simulink model "test_mdl_NI"  (R2018a)
settings: Solver=VariableStepAuto  StartTime=0.0  StopTime=10.0  RelTol=1e-3
(part 24 of 24)

== system test_mdl_NI/To_NI_HIL/SRR_L/RL_SOD/SRR_RL_002/SRR_RL_CAN_DET_RANGE_02 ==
  in : Inport
  out : Outport
  wires:
  in/1 -> out/1

== system test_mdl_NI/To_NI_HIL/SRR_L/RL_SOD/SRR_RL_002/SRR_RL_CAN_DET_RANGE_RATE_02 ==
  in : Inport
  out : Outport
  wires:
  in/1 -> out/1

== system test_mdl_NI/To_NI_HIL/SRR_L/RL_SOD/SRR_RL_002/SRR_RL_CAN_DET_SUPER_RES_TARGET_02 ==
  in : Inport
  out : Outport
  wires:
  in/1 -> out/1

== system test_mdl_NI/To_NI_HIL/SRR_L/RL_SOD/SRR_RL_002/SRR_RL_CAN_DET_VALID_LEVEL_02 ==
  in : Inport
  out : Outport
  wires:
  in/1 -> out/1

== system test_mdl_NI/To_NI_HIL/SRR_L/RL_SOD/SRR_RL_003/SRR_RL_CAN_DET_AMPLITUDE_03 ==
  in : Inport
  out : Outport
  wires:
  in/1 -> out/1

== system test_mdl_NI/To_NI_HIL/SRR_L/RL_SOD/SRR_RL_003/SRR_RL_CAN_DET_AZIMUTH_03 ==
  in : Inport
  out : Outport
  wires:
  in/1 -> out/1

== system test_mdl_NI/To_NI_HIL/SRR_L/RL_SOD/SRR_RL_003/SRR_RL_CAN_DET_ELEVATION_03 ==
  in : Inport
  out : Outport
  wires:
  in/1 -> out/1

== system test_mdl_NI/To_NI_HIL/SRR_L/RL_SOD/SRR_RL_003/SRR_RL_CAN_DET_RANGE_03 ==
  in : Inport
  out : Outport
  wires:
  in/1 -> out/1

== system test_mdl_NI/To_NI_HIL/SRR_L/RL_SOD/SRR_RL_003/SRR_RL_CAN_DET_RANGE_RATE_03 ==
  in : Inport
  out : Outport
  wires:
  in/1 -> out/1

== system test_mdl_NI/To_NI_HIL/SRR_L/RL_SOD/SRR_RL_003/SRR_RL_CAN_DET_SUPER_RES_TARGET_03 ==
  in : Inport
  out : Outport
  wires:
  in/1 -> out/1

== system test_mdl_NI/To_NI_HIL/SRR_L/RL_SOD/SRR_RL_003/SRR_RL_CAN_DET_VALID_LEVEL_03 ==
  in : Inport
  out : Outport
  wires:
  in/1 -> out/1

== system test_mdl_NI/To_NI_HIL/SRR_R/FR_SOD/SRR_FR_001/SRR_FR_CAN_DET_AMPLITUDE_01 ==
  in : Inport
  out : Outport
  wires:
  in/1 -> out/1

== system test_mdl_NI/To_NI_HIL/SRR_R/FR_SOD/SRR_FR_001/SRR_FR_CAN_DET_AZIMUTH_01 ==
  in : Inport
  out : Outport
  wires:
  in/1 -> out/1

== system test_mdl_NI/To_NI_HIL/SRR_R/FR_SOD/SRR_FR_001/SRR_FR_CAN_DET_ELEVATION_01 ==
  in : Inport
  out : Outport
  wires:
  in/1 -> out/1

== system test_mdl_NI/To_NI_HIL/SRR_R/FR_SOD/SRR_FR_001/SRR_FR_CAN_DET_RANGE_01 ==
  in : Inport
  out : Outport
  wires:
  in/1 -> out/1

== system test_mdl_NI/To_NI_HIL/SRR_R/FR_SOD/SRR_FR_001/SRR_FR_CAN_DET_RANGE_RATE_01 ==
  in : Inport
  out : Outport
  wires:
  in/1 -> out/1

== system test_mdl_NI/To_NI_HIL/SRR_R/FR_SOD/SRR_FR_001/SRR_FR_CAN_DET_SUPER_RES_TARGET_01 ==
  in : Inport
  out : Outport
  wires:
  in/1 -> out/1

== system test_mdl_NI/To_NI_HIL/SRR_R/FR_SOD/SRR_FR_001/SRR_FR_CAN_DET_VALID_LEVEL_01 ==
  in : Inport
  out : Outport
  wires:
  in/1 -> out/1

== system test_mdl_NI/To_NI_HIL/SRR_R/FR_SOD/SRR_FR_002/SRR_FR_CAN_DET_AMPLITUDE_02 ==
  in : Inport
  out : Outport
  wires:
  in/1 -> out/1

== system test_mdl_NI/To_NI_HIL/SRR_R/FR_SOD/SRR_FR_002/SRR_FR_CAN_DET_AZIMUTH_02 ==
  in : Inport
  out : Outport
  wires:
  in/1 -> out/1

== system test_mdl_NI/To_NI_HIL/SRR_R/FR_SOD/SRR_FR_002/SRR_FR_CAN_DET_ELEVATION_02 ==
  in : Inport
  out : Outport
  wires:
  in/1 -> out/1

== system test_mdl_NI/To_NI_HIL/SRR_R/FR_SOD/SRR_FR_002/SRR_FR_CAN_DET_RANGE_02 ==
  in : Inport
  out : Outport
  wires:
  in/1 -> out/1

== system test_mdl_NI/To_NI_HIL/SRR_R/FR_SOD/SRR_FR_002/SRR_FR_CAN_DET_RANGE_RATE_02 ==
  in : Inport
  out : Outport
  wires:
  in/1 -> out/1

== system test_mdl_NI/To_NI_HIL/SRR_R/FR_SOD/SRR_FR_002/SRR_FR_CAN_DET_SUPER_RES_TARGET_02 ==
  in : Inport
  out : Outport
  wires:
  in/1 -> out/1

== system test_mdl_NI/To_NI_HIL/SRR_R/FR_SOD/SRR_FR_002/SRR_FR_CAN_DET_VALID_LEVEL_02 ==
  in : Inport
  out : Outport
  wires:
  in/1 -> out/1

== system test_mdl_NI/To_NI_HIL/SRR_R/FR_SOD/SRR_FR_003/SRR_FR_CAN_DET_AMPLITUDE_03 ==
  in : Inport
  out : Outport
  wires:
  in/1 -> out/1

== system test_mdl_NI/To_NI_HIL/SRR_R/FR_SOD/SRR_FR_003/SRR_FR_CAN_DET_AZIMUTH_03 ==
  in : Inport
  out : Outport
  wires:
  in/1 -> out/1

== system test_mdl_NI/To_NI_HIL/SRR_R/FR_SOD/SRR_FR_003/SRR_FR_CAN_DET_ELEVATION_03 ==
  in : Inport
  out : Outport
  wires:
  in/1 -> out/1

== system test_mdl_NI/To_NI_HIL/SRR_R/FR_SOD/SRR_FR_003/SRR_FR_CAN_DET_RANGE_03 ==
  in : Inport
  out : Outport
  wires:
  in/1 -> out/1

== system test_mdl_NI/To_NI_HIL/SRR_R/FR_SOD/SRR_FR_003/SRR_FR_CAN_DET_RANGE_RATE_03 ==
  in : Inport
  out : Outport
  wires:
  in/1 -> out/1

== system test_mdl_NI/To_NI_HIL/SRR_R/FR_SOD/SRR_FR_003/SRR_FR_CAN_DET_SUPER_RES_TARGET_03 ==
  in : Inport
  out : Outport
  wires:
  in/1 -> out/1

== system test_mdl_NI/To_NI_HIL/SRR_R/FR_SOD/SRR_FR_003/SRR_FR_CAN_DET_VALID_LEVEL_03 ==
  in : Inport
  out : Outport
  wires:
  in/1 -> out/1

== system test_mdl_NI/To_NI_HIL/SRR_R/RR_SOD/SRR_RR_001/SRR_RR_CAN_DET_AMPLITUDE_01 ==
  in : Inport
  out : Outport
  wires:
  in/1 -> out/1

== system test_mdl_NI/To_NI_HIL/SRR_R/RR_SOD/SRR_RR_001/SRR_RR_CAN_DET_AZIMUTH_01 ==
  in : Inport
  out : Outport
  wires:
  in/1 -> out/1

== system test_mdl_NI/To_NI_HIL/SRR_R/RR_SOD/SRR_RR_001/SRR_RR_CAN_DET_ELEVATION_01 ==
  in : Inport
  out : Outport
  wires:
  in/1 -> out/1

== system test_mdl_NI/To_NI_HIL/SRR_R/RR_SOD/SRR_RR_001/SRR_RR_CAN_DET_RANGE_01 ==
  in : Inport
  out : Outport
  wires:
  in/1 -> out/1

== system test_mdl_NI/To_NI_HIL/SRR_R/RR_SOD/SRR_RR_001/SRR_RR_CAN_DET_RANGE_RATE_01 ==
  in : Inport
  out : Outport
  wires:
  in/1 -> out/1

== system test_mdl_NI/To_NI_HIL/SRR_R/RR_SOD/SRR_RR_001/SRR_RR_CAN_DET_SUPER_RES_TARGET_01 ==
  in : Inport
  out : Outport
  wires:
  in/1 -> out/1

== system test_mdl_NI/To_NI_HIL/SRR_R/RR_SOD/SRR_RR_001/SRR_RR_CAN_DET_VALID_LEVEL_01 ==
  in : Inport
  out : Outport
  wires:
  in/1 -> out/1

== system test_mdl_NI/To_NI_HIL/SRR_R/RR_SOD/SRR_RR_002/SRR_RR_CAN_DET_AMPLITUDE_02 ==
  in : Inport
  out : Outport
  wires:
  in/1 -> out/1

== system test_mdl_NI/To_NI_HIL/SRR_R/RR_SOD/SRR_RR_002/SRR_RR_CAN_DET_AZIMUTH_02 ==
  in : Inport
  out : Outport
  wires:
  in/1 -> out/1

== system test_mdl_NI/To_NI_HIL/SRR_R/RR_SOD/SRR_RR_002/SRR_RR_CAN_DET_ELEVATION_02 ==
  in : Inport
  out : Outport
  wires:
  in/1 -> out/1

== system test_mdl_NI/To_NI_HIL/SRR_R/RR_SOD/SRR_RR_002/SRR_RR_CAN_DET_RANGE_02 ==
  in : Inport
  out : Outport
  wires:
  in/1 -> out/1

== system test_mdl_NI/To_NI_HIL/SRR_R/RR_SOD/SRR_RR_002/SRR_RR_CAN_DET_RANGE_RATE_02 ==
  in : Inport
  out : Outport
  wires:
  in/1 -> out/1

== system test_mdl_NI/To_NI_HIL/SRR_R/RR_SOD/SRR_RR_002/SRR_RR_CAN_DET_SUPER_RES_TARGET_02 ==
  in : Inport
  out : Outport
  wires:
  in/1 -> out/1

== system test_mdl_NI/To_NI_HIL/SRR_R/RR_SOD/SRR_RR_002/SRR_RR_CAN_DET_VALID_LEVEL_02 ==
  in : Inport
  out : Outport
  wires:
  in/1 -> out/1

== system test_mdl_NI/To_NI_HIL/SRR_R/RR_SOD/SRR_RR_003/SRR_RR_CAN_DET_AMPLITUDE_03 ==
  in : Inport
  out : Outport
  wires:
  in/1 -> out/1

== system test_mdl_NI/To_NI_HIL/SRR_R/RR_SOD/SRR_RR_003/SRR_RR_CAN_DET_AZIMUTH_03 ==
  in : Inport
  out : Outport
  wires:
  in/1 -> out/1

== system test_mdl_NI/To_NI_HIL/SRR_R/RR_SOD/SRR_RR_003/SRR_RR_CAN_DET_ELEVATION_03 ==
  in : Inport
  out : Outport
  wires:
  in/1 -> out/1

== system test_mdl_NI/To_NI_HIL/SRR_R/RR_SOD/SRR_RR_003/SRR_RR_CAN_DET_RANGE_03 ==
  in : Inport
  out : Outport
  wires:
  in/1 -> out/1

== system test_mdl_NI/To_NI_HIL/SRR_R/RR_SOD/SRR_RR_003/SRR_RR_CAN_DET_RANGE_RATE_03 ==
  in : Inport
  out : Outport
  wires:
  in/1 -> out/1

== system test_mdl_NI/To_NI_HIL/SRR_R/RR_SOD/SRR_RR_003/SRR_RR_CAN_DET_SUPER_RES_TARGET_03 ==
  in : Inport
  out : Outport
  wires:
  in/1 -> out/1

== system test_mdl_NI/To_NI_HIL/SRR_R/RR_SOD/SRR_RR_003/SRR_RR_CAN_DET_VALID_LEVEL_03 ==
  in : Inport
  out : Outport
  wires:
  in/1 -> out/1

== system test_mdl_NI/To_NI_HIL/Soft_MRR/MRR_Detection/MRR_Detection_001/CAN_DET_AMPLITUDE_01 ==
  in : Inport
  out : Outport
  wires:
  in/1 -> out/1

== system test_mdl_NI/To_NI_HIL/Soft_MRR/MRR_Detection/MRR_Detection_001/CAN_DET_AZIMUTH_01 ==
  in : Inport
  out : Outport
  wires:
  in/1 -> out/1

== system test_mdl_NI/To_NI_HIL/Soft_MRR/MRR_Detection/MRR_Detection_001/CAN_DET_RANGE_01 ==
  in : Inport
  out : Outport
  wires:
  in/1 -> out/1

== system test_mdl_NI/To_NI_HIL/Soft_MRR/MRR_Detection/MRR_Detection_001/CAN_DET_RANGE_RATE_01 ==
  in : Inport
  out : Outport
  wires:
  in/1 -> out/1

== system test_mdl_NI/To_NI_HIL/Soft_MRR/MRR_Detection/MRR_Detection_001/CAN_DET_VALID_LEVEL_01 ==
  in : Inport
  out : Outport
  wires:
  in/1 -> out/1

== system test_mdl_NI/To_NI_HIL/Soft_MRR/MRR_Detection/MRR_Detection_002/CAN_DET_AMPLITUDE_02 ==
  in : Inport
  out : Outport
  wires:
  in/1 -> out/1

== system test_mdl_NI/To_NI_HIL/Soft_MRR/MRR_Detection/MRR_Detection_002/CAN_DET_AZIMUTH_02 ==
  in : Inport
  out : Outport
  wires:
  in/1 -> out/1

== system test_mdl_NI/To_NI_HIL/Soft_MRR/MRR_Detection/MRR_Detection_002/CAN_DET_RANGE_02 ==
  in : Inport
  out : Outport
  wires:
  in/1 -> out/1

== system test_mdl_NI/To_NI_HIL/Soft_MRR/MRR_Detection/MRR_Detection_002/CAN_DET_RANGE_RATE_02 ==
  in : Inport
  out : Outport
  wires:
  in/1 -> out/1

== system test_mdl_NI/To_NI_HIL/Soft_MRR/MRR_Detection/MRR_Detection_002/CAN_DET_VALID_LEVEL_02 ==
  in : Inport
  out : Outport
  wires:
  in/1 -> out/1

== system test_mdl_NI/To_NI_HIL/Soft_MRR/MRR_Detection/MRR_Detection_003/CAN_DET_AMPLITUDE_03 ==
  in : Inport
  out : Outport
  wires:
  in/1 -> out/1

== system test_mdl_NI/To_NI_HIL/Soft_MRR/MRR_Detection/MRR_Detection_003/CAN_DET_AZIMUTH_03 ==
  in : Inport
  out : Outport
  wires:
  in/1 -> out/1

== system test_mdl_NI/To_NI_HIL/Soft_MRR/MRR_Detection/MRR_Detection_003/CAN_DET_RANGE_03 ==
  in : Inport
  out : Outport
  wires:
  in/1 -> out/1

== system test_mdl_NI/To_NI_HIL/Soft_MRR/MRR_Detection/MRR_Detection_003/CAN_DET_RANGE_RATE_03 ==
  in : Inport
  out : Outport
  wires:
  in/1 -> out/1

== system test_mdl_NI/To_NI_HIL/Soft_MRR/MRR_Detection/MRR_Detection_003/CAN_DET_VALID_LEVEL_03 ==
  in : Inport
  out : Outport
  wires:
  in/1 -> out/1
